simulink model "perturb_observe"  (R2021a)
settings: Solver=VariableStepAuto  StartTime=0.0  StopTime=5  RelTol=1e-3
undefined symbols (not defined in the file): Ts_Control, Ts_Power
libraries: spsControlledVoltageSourceLib x2, spsSeriesRLCBranchLib x2, spsPVArrayLib x1, spsControlledCurrentSourceLib x1, spsCurrentMeasurementLib x1, spsVoltageMeasurementLib x1, spsDiodeLib x1, spsStairGeneratorLib x1, spspowerguiLib x1
settings Model: Creator=shekh  LastModifiedBy=shekh

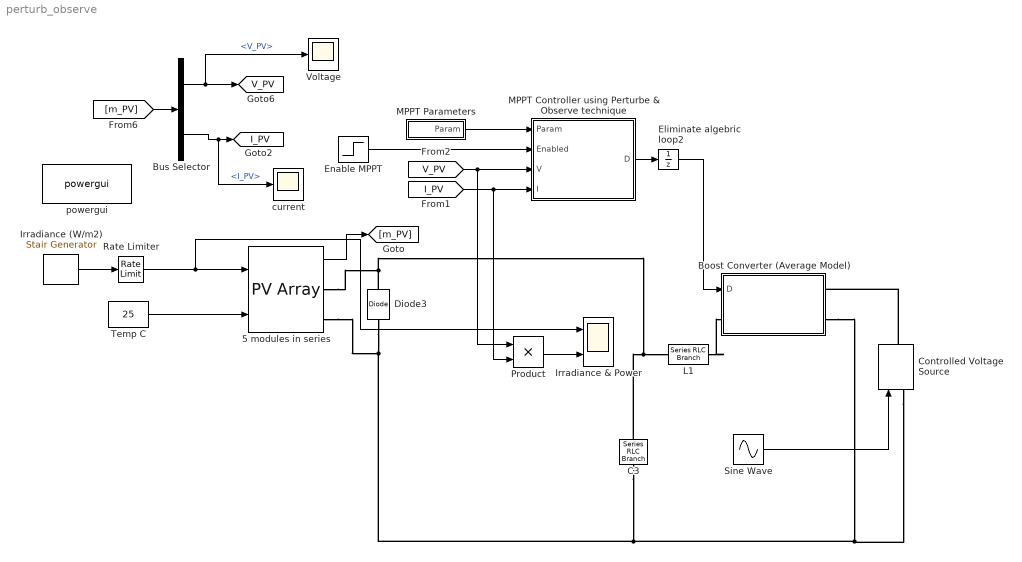
== system perturb_observe ==
  5 modules in series : spsPVArrayLib/PV Array  Npar=1  Nser=5  PlotType=array @ 25 deg.C & specified irradiances  S_vec="[1000  1000 1000 1000 400]"  Temp_C_vec=[25 25 25 25 25]  ModuleName=User-defined  PlotWhenSelected=off  Pm=215.46  Ncell=72  Voc=51.6  Isc=5.61  Vm=42  Im=5.13  beta_Voc_pc=-0.143  alpha_Isc_pc=1.96e-3  beta_Voc=-0.073788  alpha_Isc=0.00010996  IL=5.6441  I0=3.2641e-15  nI=0.79656  Rsh=146.1919  Rs=0.92078  RobustModel=off  RobustCellTemperature=313.3991  BAL=off  Tc=Tc  Tfilter=5e-5
  Boost Converter (Average Model) : Subsystem  mask(Boost Converter (Average Model)){Ts=Ts_Power}
      mask prompts: Ts "Sample time:"
      mask Display: disp('Boost\n(Average)')
  Bus Selector : BusSelector  OutputSignals=V_PV,I_PV
  C3 : spsSeriesRLCBranchLib/Series RLC Branch  LConnTagsString=__new0  RConnTagsString=__new0  BranchType=C  Resistance=1.0  Inductance=1.0  SetiL0=off  InitialCurrent=0  Capacitance=100e-6  Setx0=off  InitialVoltage=0  Measurements=Branch voltage
  Controlled Voltage Source : spsControlledVoltageSourceLib/Controlled Voltage Source  Initialize=on  Source_Type=DC  Amplitude=500  Phase=0  Frequency=0  Measurements=None
  Diode3 : spsDiodeLib/Diode  Ron=0.001  Lon=0  Vf=0.7  IC=0  UseSnubber=off  Rs=1e5*inf  Cs=inf  Measurements=off
  Eliminate algebric loop2 : UnitDelay  SampleTime=Ts_Control  HasFrameUpgradeWarning=on
  Enable MPPT : Step  Time=0.25  SampleTime=0
  Irradiance & Power : Scope  NumInputPorts=2
  Irradiance (W/m2) : spsStairGeneratorLib/Stair Generator  t=[1, 1.6, 1.8, 1.9,3]  e=[1/2, 1/2, 1/2, 1/2,1/2]*1000  Ts=Ts_Power
  L1 : spsSeriesRLCBranchLib/Series RLC Branch  LConnTagsString=__new0  RConnTagsString=__new0  BranchType=RL  Resistance=0.005  Inductance=5e-3  SetiL0=off  InitialCurrent=0  Capacitance=1e-6  Setx0=off  InitialVoltage=0  Measurements=None
  MPPT Parameters : Subsystem
  "MPPT Controller using Perturbe & Observe technique " : MATLAB Function  TreatAsAtomicUnit=on
  Product : Product
  Rate Limiter : RateLimiter  RisingSlewLimit=6000  FallingSlewLimit=-6000  SampleTimeMode=inherited  InitialCondition=1000
  Sine Wave : Sin  Amplitude=0.1  Bias=400  Frequency=2*pi  SampleTime=0
  Temp C : Constant  Value=25
  Voltage : Scope
  current : Scope
  powergui : spspowerguiLib/powergui  Priority=1  SimulationMode=Continuous  SampleTime=Ts_Power  frequency=60  Iterations=50  frequencyindice=0  Pbase=100e6  ErrMax=1e-4  UnitsV=kV  UnitsW=MW  buscounter=0  FunctionMessages=off  echomessages=off  EnableUseOfTLC=off  CurrentSourceSwitches=off  DisableSnubberDevices=off  DisableRonSwitches=off  DisableVfSwitches=off  DisplayEquations=off  AutomaticDiscreteSolvers=off  SolverType=Tustin/Backward Euler (TBE)  Interpol=off  ExternalGateDelay=off  methode=off  Ts=0  x0status=blocks  SPID=off  SwTol=0  HookPort=off  NonlinearTolerance=1e-4  nMaxIteration=100  ContinueOnMaxIteration=off  RestoreLinks=warning  ResistiveCurrentMeasurement=off  Frange=[0:2:500]  Ylog=off  Xlog=on  ShowGrid=off  save=off  variable=ZData  structure=0  ZoomFFT=on  StartTime=0.0  cycles=1  DisplayStyle=1  fundamental=60  FreqAxis=off  MaxFrequency=1000  frequencyindicesteady=1  RmsSteady=1  display=off
  tag scope: I_PV=global, V_PV=global
  wires:
  Sine Wave/1 -> Controlled Voltage Source/1
  Bus Selector/2 -> current/1, [I_PV]  "<I_PV>"
  Bus Selector/1 -> Voltage/1, [V_PV]  "<V_PV>"
  Rate Limiter/1 -> Irradiance & Power/1, 5 modules in series/1
  Irradiance (W/m2)/1 -> Rate Limiter/1
  [I_PV] -> Product/2, "MPPT Controller using Perturbe & Observe technique "/4(I)
  [V_PV] -> Product/1, "MPPT Controller using Perturbe & Observe technique "/3(V)
  MPPT Parameters/1(Param) -> "MPPT Controller using Perturbe & Observe technique "/1(Param)
  [m_PV] -> Bus Selector/1
  Eliminate algebric loop2/1 -> Boost Converter (Average Model)/1(D)
  Enable MPPT/1 -> "MPPT Controller using Perturbe & Observe technique "/2(Enabled)
  Product/1 -> Irradiance & Power/2
  Temp C/1 -> 5 modules in series/2
  "MPPT Controller using Perturbe & Observe technique "/1(D) -> Eliminate algebric loop2/1
  5 modules in series/1 -> [m_PV]
  connections:
  5 modules in series/RConn2 -- C3/RConn1 -- Boost Converter (Average Model)/RConn2 -- Controlled Voltage Source/LConn1 -- Diode3/LConn1
  5 modules in series/RConn1 -- Diode3/RConn1 -- C3/LConn1 -- L1/LConn1
  Controlled Voltage Source/RConn1 -- Boost Converter (Average Model)/RConn1
  L1/RConn1 -- Boost Converter (Average Model)/LConn1

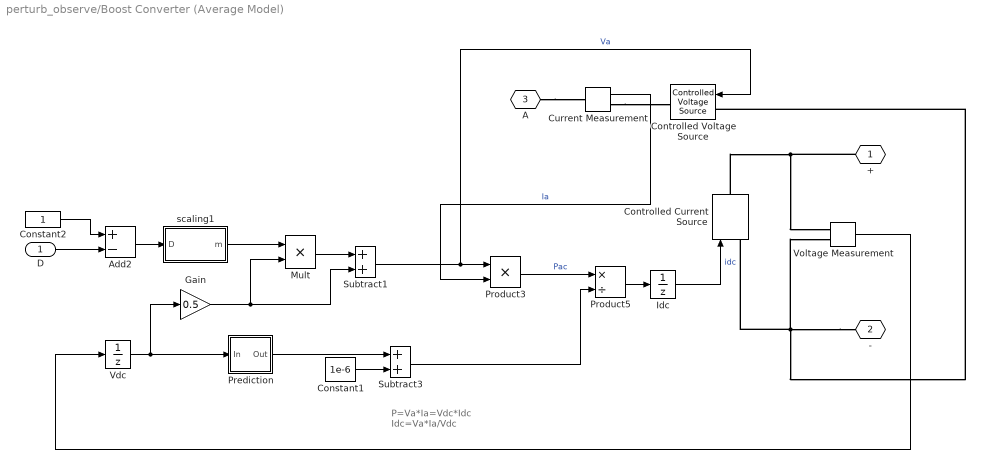
== system perturb_observe/Boost Converter (Average Model) ==
  note: P=Va*Ia=Vdc*Idc
      | Idc=Va*Ia/Vdc
  D : Inport
  Add2 : Sum  Inputs=+-
  Constant1 : Constant  Value=1e-6
  Constant2 : Constant
  Controlled Current Source : spsControlledCurrentSourceLib/Controlled Current Source  Initialize=on  Source_Type=AC  Amplitude=0  Phase=0  Frequency=0  Measurements=None
  Controlled Voltage Source : spsControlledVoltageSourceLib/Controlled Voltage Source  Initialize=on  Source_Type=AC  Amplitude=0  Phase=0  Frequency=0  Measurements=None
  Current Measurement : spsCurrentMeasurementLib/Current Measurement  PhasorSimulation=off  OutputType=Complex  PSBequivalent=0
  Gain : Gain  Gain=0.5
  Idc : UnitDelay  SampleTime=Ts  HasFrameUpgradeWarning=on
  Mult : Product  Inputs=**
  Prediction : Subsystem
  Product3 : Product  RndMeth=Zero
  Product5 : Product  Inputs=*/  RndMeth=Zero
  Subtract1 : Sum
  Subtract3 : Sum
  Vdc : UnitDelay  SampleTime=Ts  HasFrameUpgradeWarning=on
  Voltage Measurement : spsVoltageMeasurementLib/Voltage Measurement  PhasorSimulation=off  OutputType=Complex  PSBequivalent=0
  scaling1 : Subsystem
  + : PMIOPort  Tag=PMCPort  Side=Right
  - : PMIOPort  Tag=PMCPort  Port=2  Side=Right
  A : PMIOPort  Tag=PMCPort  Port=3  Side=Left
  wires:
  Gain/1 -> Mult/2, Subtract1/2
  Product5/1 -> Idc/1
  Constant1/1 -> Subtract3/2
  Subtract3/1 -> Product5/2
  Product3/1 -> Product5/1  "Pac"
  Prediction/1(Out) -> Subtract3/1
  Vdc/1 -> Prediction/1(In), Gain/1
  Subtract1/1 -> Product3/1, Controlled Voltage Source/1  "Va"
  Mult/1 -> Subtract1/1
  Constant2/1 -> Add2/1
  Add2/1 -> scaling1/1(D)
  scaling1/1(m) -> Mult/1
  D/1 -> Add2/2
  Voltage Measurement/1 -> Vdc/1
  Idc/1 -> Controlled Current Source/1  "idc"
  Current Measurement/1 -> Product3/2  "Ia"
  connections:
  -/RConn1 -- Voltage Measurement/LConn2 -- Controlled Voltage Source/LConn1 -- Controlled Current Source/LConn1
  +/RConn1 -- Voltage Measurement/LConn1 -- Controlled Current Source/RConn1
  Current Measurement/RConn1 -- Controlled Voltage Source/RConn1
  A/RConn1 -- Current Measurement/LConn1

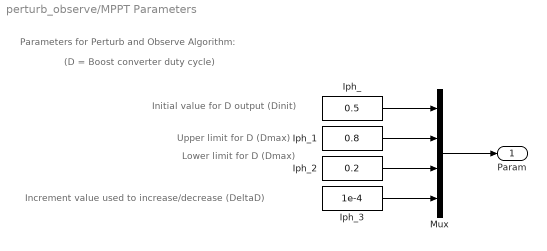
== system perturb_observe/MPPT Parameters ==
  note: Upper limit for D (Dmax)
  note: Increment value used to increase/decrease (DeltaD)
  note: Initial value for D output (Dinit)
  note: (D = Boost converter duty cycle)
  note: Lower limit for D (Dmax)
  note: Parameters for Perturb and Observe Algorithm:
  Iph_ : Constant  Value=0.5
  Iph_1 : Constant  Value=0.8
  Iph_2 : Constant  Value=0.2
  Iph_3 : Constant  Value=1e-4
  Mux : Mux
  Param : Outport
  wires:
  Iph_/1 -> Mux/1
  Iph_1/1 -> Mux/2
  Iph_2/1 -> Mux/3
  Iph_3/1 -> Mux/4
  Mux/1 -> Param/1

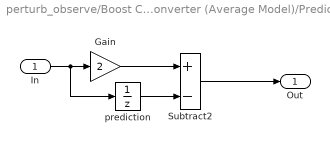
== system perturb_observe/Boost Converter (Average Model)/Prediction ==
  In : Inport
  Gain : Gain  Gain=2
  Subtract2 : Sum  Inputs=+-
  prediction : UnitDelay  SampleTime=Ts  HasFrameUpgradeWarning=on
  Out : Outport
  wires:
  prediction/1 -> Subtract2/2
  In/1 -> prediction/1, Gain/1
  Subtract2/1 -> Out/1
  Gain/1 -> Subtract2/1

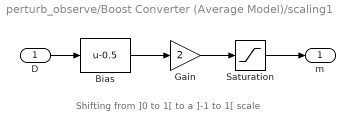
== system perturb_observe/Boost Converter (Average Model)/scaling1 ==
  note: Shifting from ]0 to 1[ to a ]-1 to 1[ scale
  D : Inport
  Bias : Bias  Bias=-0.5
  Gain : Gain  Gain=2
  Saturation : Saturate  UpperLimit=1  LowerLimit=-1
  m : Outport
  wires:
  Saturation/1 -> m/1
  Gain/1 -> Saturation/1
  D/1 -> Bias/1
  Bias/1 -> Gain/1

== matlab function perturb_observe/MPPT Controller using Perturbe & Observe technique  ==
  settings: updateMethod=DISCRETE  sampleTime=Ts_Control
  data: Param input; Enabled input; V input =V; I input; D output
function D  = PandO(Param, Enabled, V, I)

% MPPT controller based on the Perturb & Observe algorithm.

% D output = Duty cycle of the boost converter (value between 0 and 1)
%
% Enabled input = 1 to enable the MPPT controller
% V input = PV array terminal voltage (V)
% I input = PV array current (A)
%
% Param input:
Dinit = Param(1);  %Initial value for D output
Dmax = Param(2);   %Maximum value for D
Dmin = Param(3);   %Minimum value for D
deltaD = Param(4); %Increment value used to increase/decrease the duty cycle D
% ( increasing D = decreasing Vref )
%  

persistent Vold Pold Dold;

dataType = 'double';

if isempty(Vold)
    Vold=0;
    Pold=0;
    Dold=Dinit;
end
P= V*I;
dV= V - Vold;
dP= P - Pold;

if dP ~= 0 & Enabled ~=0
    if dP < 0
        if dV < 0
            D = Dold - deltaD;
        else
            D = Dold + deltaD;
        end
    else
        if dV < 0
            D = Dold + deltaD;
        else
            D = Dold - deltaD;
        end    
    end
else D=Dold;
end

if D >= Dmax | D<= Dmin
    D=Dold;
end

Dold=D;
Vold=V;
Pold=P;
